simulink model "TP3_synchrone"  (R2017b)
settings: Solver=ode23t  StartTime=0.0  StopTime=30  RelTol=1e-3
InitFcn:
  | TP3_config
values from neighbouring files (symbols this model uses):
  J = 0.2    [TP3_config.m]
  K = 0.9    [TP3_config.m]
  L = 12.161e-3    (= 0.012161)    [TP3_config.m]
  p = 3    [TP3_config.m]
  R = 0.895    [TP3_config.m]
settings Model: Creator=GEII Robot  LastModifiedBy=GEII Robot

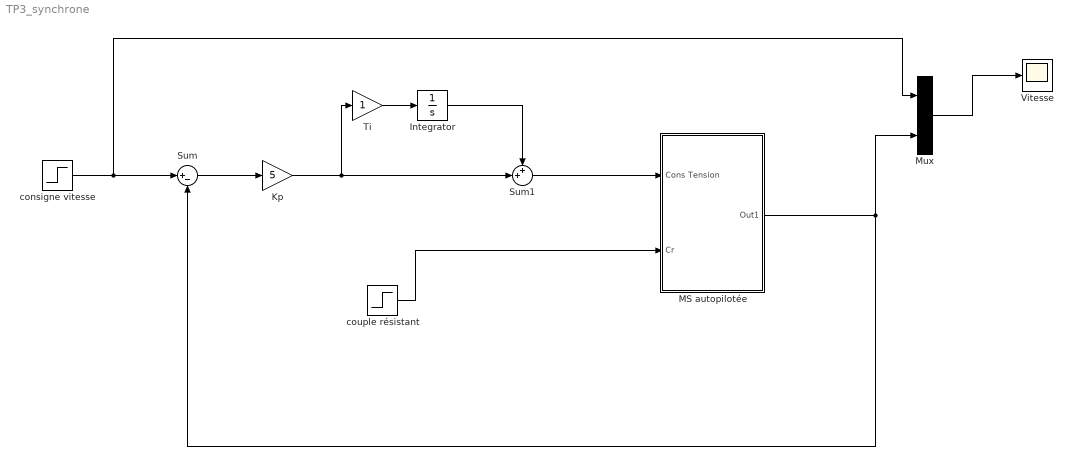
== system TP3_synchrone ==
  Integrator : Integrator
  "Kp " : Gain  Gain=5
  MS autopilotée : Subsystem
  Mux : Mux  Inputs=2
  Sum : Sum  Inputs=|+-
  Sum1 : Sum  Inputs=++|
  "Ti " : Gain
  Vitesse : Scope
  consigne vitesse : Step  Time=0  After=10  SampleTime=0
  couple résistant : Step  Time=3  After=20  SampleTime=0
  wires:
  couple résistant/1 -> MS autopilotée/2(Cr)
  Sum1/1 -> MS autopilotée/1(Cons Tension)
  Integrator/1 -> Sum1/1
  "Kp "/1 -> "Ti "/1, Sum1/2
  "Ti "/1 -> Integrator/1
  Sum/1 -> "Kp "/1
  consigne vitesse/1 -> Mux/1, Sum/1
  Mux/1 -> Vitesse/1
  MS autopilotée/1(Out1) -> Mux/2, Sum/2

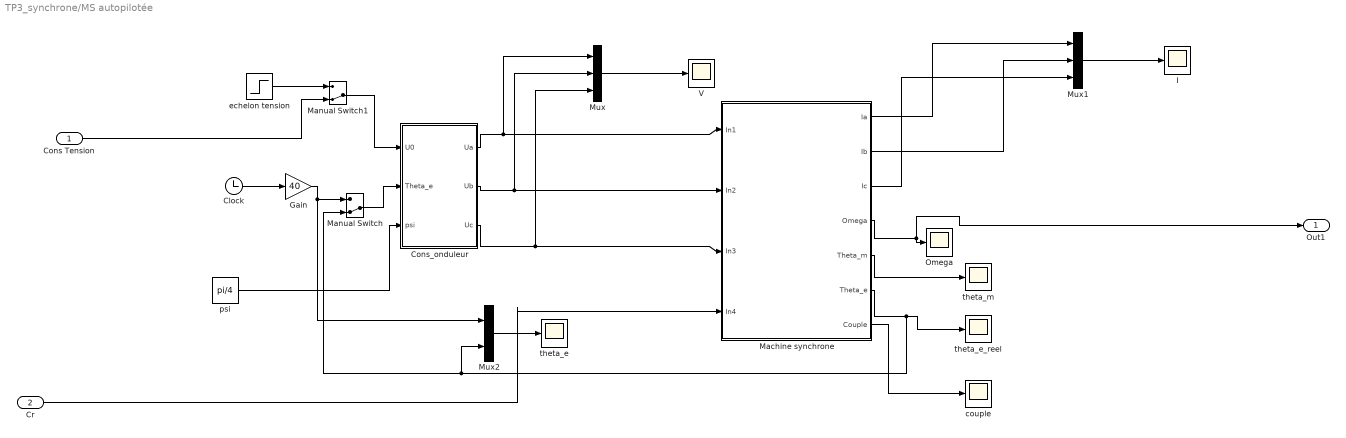
== system TP3_synchrone/MS autopilotée ==
  Cons Tension : Inport
  Cr : Inport  Port=2
  Clock : Clock
  "Cons_onduleur " : Subsystem
  Gain : Gain  Gain=40
  I : Scope
  Machine synchrone : Subsystem
  Manual Switch : ManualSwitch  CurrentSetting=0
  Manual Switch1 : ManualSwitch  CurrentSetting=0
  Mux : Mux  Inputs=3
  Mux1 : Mux  Inputs=3
  Mux2 : Mux  Inputs=2
  Omega : Scope
  V : Scope
  couple : Scope
  echelon tension : Step  Time=0  SampleTime=0
  psi : Constant  Value=pi/4
  theta_e : Scope
  theta_e_reel : Scope
  theta_m : Scope
  Out1 : Outport
  wires:
  Machine synchrone/7(Couple) -> couple/1
  Cons Tension/1 -> Manual Switch1/2
  echelon tension/1 -> Manual Switch1/1
  Manual Switch1/1 -> "Cons_onduleur "/1(U0)
  Cr/1 -> Machine synchrone/4(In4)
  Machine synchrone/4(Omega) -> Out1/1, Omega/1
  Machine synchrone/5(Theta_m) -> theta_m/1
  Machine synchrone/2(Ib) -> Mux1/2
  Mux/1 -> V/1
  Machine synchrone/3(Ic) -> Mux1/3
  Mux1/1 -> I/1
  Gain/1 -> Manual Switch/1, Mux2/1
  "Cons_onduleur "/2(Ub) -> Mux/2, Machine synchrone/2(In2)
  psi/1 -> "Cons_onduleur "/3(psi)
  "Cons_onduleur "/1(Ua) -> Mux/1, Machine synchrone/1(In1)
  Machine synchrone/1(Ia) -> Mux1/1
  Manual Switch/1 -> "Cons_onduleur "/2(Theta_e)
  Machine synchrone/6("Theta_e ") -> Mux2/2, Manual Switch/2, theta_e_reel/1
  "Cons_onduleur "/3(Uc) -> Mux/3, Machine synchrone/3(In3)
  Clock/1 -> Gain/1
  Mux2/1 -> theta_e/1

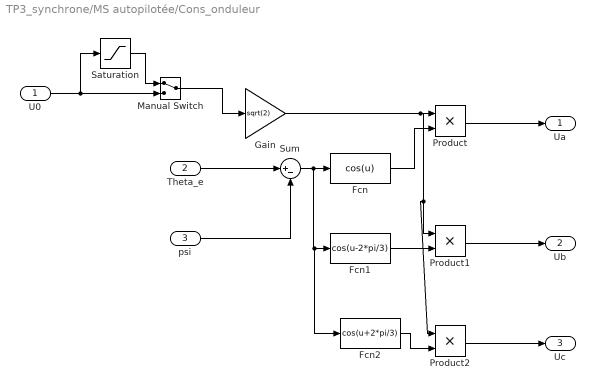
== system TP3_synchrone/MS autopilotée/Cons_onduleur  ==
  U0 : Inport
  Theta_e : Inport  Port=2
  psi : Inport  Port=3
  Fcn : Fcn  Expr=cos(u)
  Fcn1 : Fcn  Expr=cos(u-2*pi/3)
  Fcn2 : Fcn  Expr=cos(u+2*pi/3)
  Gain : Gain  Gain=sqrt(2)
  Manual Switch : ManualSwitch
  Product : Product
  Product1 : Product
  Product2 : Product
  Saturation : Saturate  UpperLimit=220  LowerLimit=-220
  Sum : Sum  Inputs=|+-
  Ua : Outport
  Ub : Outport  Port=2
  Uc : Outport  Port=3
  wires:
  Product/1 -> Ua/1
  Theta_e/1 -> Sum/1
  psi/1 -> Sum/2
  Fcn/1 -> Product/2
  Gain/1 -> Product2/1, Product1/1, Product/1
  Product2/1 -> Uc/1
  Fcn1/1 -> Product1/2
  Product1/1 -> Ub/1
  Sum/1 -> Fcn2/1, Fcn1/1, Fcn/1
  Fcn2/1 -> Product2/2
  Manual Switch/1 -> Gain/1
  Saturation/1 -> Manual Switch/1
  U0/1 -> Saturation/1, Manual Switch/2

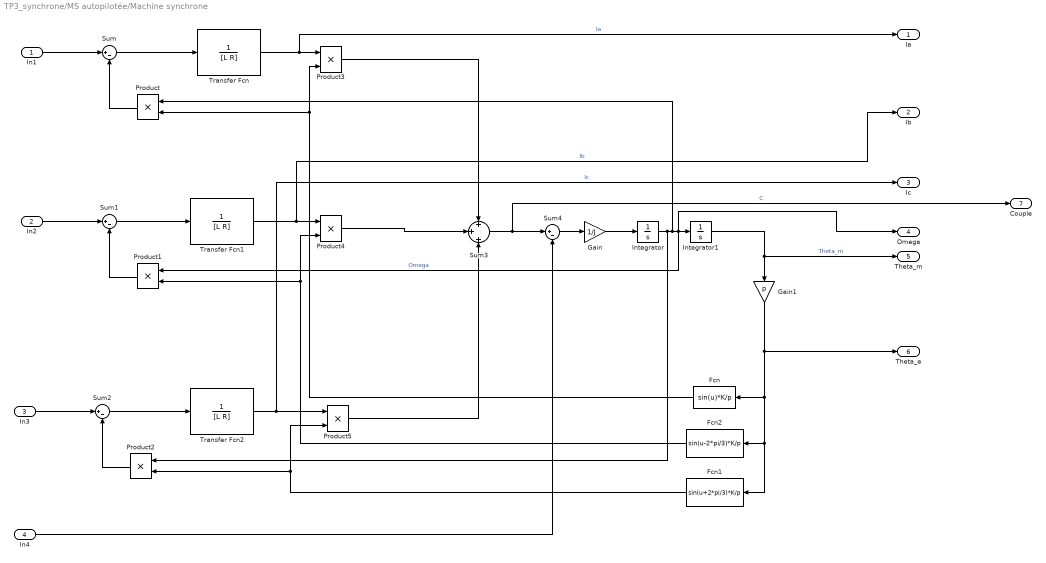
== system TP3_synchrone/MS autopilotée/Machine synchrone ==
  In1 : Inport
  In2 : Inport  Port=2
  In3 : Inport  Port=3
  In4 : Inport  Port=4
  Fcn : Fcn  Expr=sin(u)*K/p
  Fcn1 : Fcn  Expr=sin(u+2*pi/3)*K/p
  Fcn2 : Fcn  Expr=sin(u-2*pi/3)*K/p
  Gain : Gain  Gain=1/J
  Gain1 : Gain  Gain=p
  Integrator : Integrator
  Integrator1 : Integrator
  Product{,1..5} (6 alike) : Product
  Sum{,1..2,4} (4 alike) : Sum  Inputs=|+-
  Sum3 : Sum  Inputs=+|+|+
  Transfer Fcn : TransferFcn  Denominator=[L R]
  Transfer Fcn1 : TransferFcn  Denominator=[L R]
  Transfer Fcn2 : TransferFcn  Denominator=[L R]
  Ia : Outport
  Ib : Outport  Port=2
  Ic : Outport  Port=3
  Omega : Outport  Port=4
  Theta_m : Outport  Port=5
  "Theta_e " : Outport  Port=6
  Couple : Outport  Port=7
  wires:
  Transfer Fcn/1 -> Ia/1, Product3/1  "Ia"
  Sum/1 -> Transfer Fcn/1
  Fcn1/1 -> Product2/2, Product5/2
  Gain/1 -> Integrator/1
  Product1/1 -> Sum1/2
  Sum1/1 -> Transfer Fcn1/1
  Product5/1 -> Sum3/3
  Gain1/1 -> "Theta_e "/1, Fcn1/1, Fcn2/1, Fcn/1
  Fcn2/1 -> Product1/2, Product4/2
  In1/1 -> Sum/1
  Transfer Fcn1/1 -> Ib/1, Product4/1  "Ib"
  Sum2/1 -> Transfer Fcn2/1
  In3/1 -> Sum2/1
  Product2/1 -> Sum2/2
  Product/1 -> Sum/2
  Sum3/1 -> Couple/1, Sum4/1  "C"
  In2/1 -> Sum1/1
  Sum4/1 -> Gain/1
  Fcn/1 -> Product/2, Product3/2
  Integrator/1 -> Product2/1, Product/1, Omega/1, Product1/1, Integrator1/1  "Omega"
  Transfer Fcn2/1 -> Ic/1, Product5/1  "Ic"
  Integrator1/1 -> Theta_m/1, Gain1/1  "Theta_m"
  Product3/1 -> Sum3/1
  Product4/1 -> Sum3/2
  In4/1 -> Sum4/2
